simulink model "zad_no_10"  (R2017b)
settings: Solver=VariableStepAuto  StartTime=0.0  StopTime=40  RelTol=1e-3
undefined symbols (not defined in the file): Tp, u_c
settings Model: Creator=micha  LastModifiedBy=micha

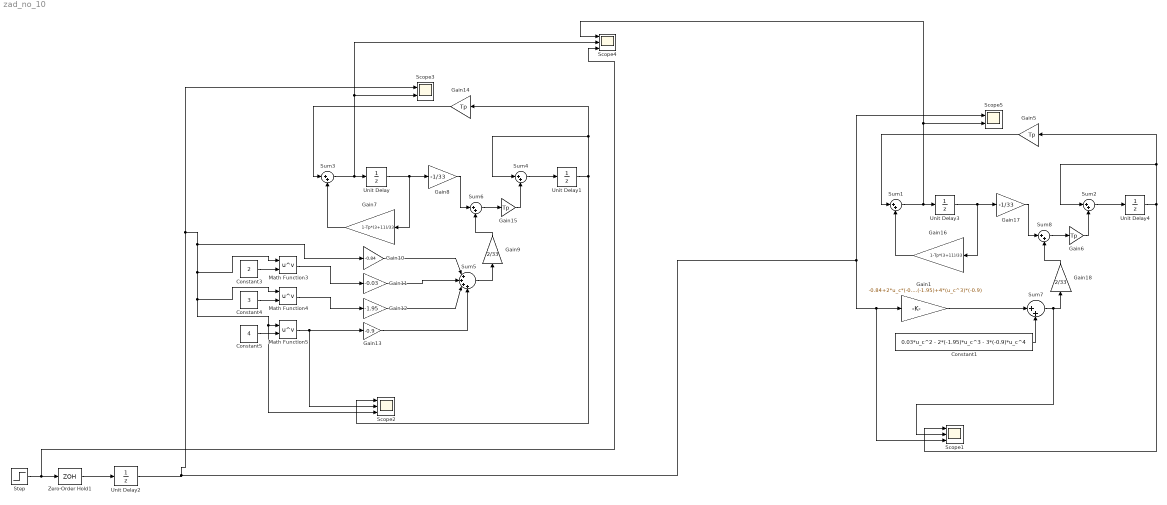
== system zad_no_10 ==
  Constant1 : Constant  Value=0.03*u_c^2 - 2*(-1.95)*u_c^3 - 3*(-0.9)*u_c^4
  Constant3 : Constant  Value=2
  Constant4 : Constant  Value=3
  Constant5 : Constant  Value=4
  Gain1 : Gain  Gain=-0.84+2*u_c*(-0.03)+3*(u_c^2)*(-1.95)+4*(u_c^3)*(-0.9)
  Gain10 : Gain  Gain=-0.84
  Gain11 : Gain  Gain=-0.03
  Gain12 : Gain  Gain=-1.95
  Gain13 : Gain  Gain=-0.9
  Gain14 : Gain  Gain=Tp  ParamDataTypeStr=double
  Gain15 : Gain  Gain=Tp
  Gain16 : Gain  Gain=1-Tp*(3+11)/33  ParamDataTypeStr=double
  Gain17 : Gain  Gain=-1/33
  Gain18 : Gain  Gain=2/33
  Gain5 : Gain  Gain=Tp  ParamDataTypeStr=double
  Gain6 : Gain  Gain=Tp
  Gain7 : Gain  Gain=1-Tp*(3+11)/33  ParamDataTypeStr=double
  Gain8 : Gain  Gain=-1/33
  Gain9 : Gain  Gain=2/33
  Math Function3 : Math  Operator=pow  SaturateOnIntegerOverflow=on
  Math Function4 : Math  Operator=pow  SaturateOnIntegerOverflow=on
  Math Function5 : Math  Operator=pow  SaturateOnIntegerOverflow=on
  Scope1 : Scope  NumInputPorts=3
  Scope2 : Scope  NumInputPorts=3
  Scope3 : Scope  NumInputPorts=2
  Scope4 : Scope  NumInputPorts=3
  Scope5 : Scope  NumInputPorts=2
  Step : Step  SampleTime=0
  Sum{1..4,6..8} (7 alike) : Sum  Inputs=|++
  Sum5 : Sum  Inputs=|++++
  Unit Delay{,1..4} (5 alike) : UnitDelay  SampleTime=Tp
  Zero-Order Hold1 : ZeroOrderHold  SampleTime=Tp
  wires:
  Sum4/1 -> Unit Delay1/1
  Constant5/1 -> Math Function5/2
  Gain7/1 -> Sum3/2
  Unit Delay/1 -> Gain8/1, Gain7/1
  Math Function5/1 -> Scope2/2, Gain13/1
  Gain10/1 -> Sum5/1
  Constant4/1 -> Math Function4/2
  Math Function4/1 -> Gain12/1
  Math Function3/1 -> Gain11/1
  Sum3/1 -> Scope3/2, Scope4/2, Unit Delay/1
  Gain12/1 -> Sum5/3
  Gain11/1 -> Sum5/2
  Unit Delay1/1 -> Sum4/1, Gain14/1, Scope2/1
  Constant3/1 -> Math Function3/2
  Gain13/1 -> Sum5/4
  Sum5/1 -> Gain9/1
  Gain14/1 -> Sum3/1
  Gain9/1 -> Sum6/2
  Gain8/1 -> Sum6/1
  Sum6/1 -> Gain15/1
  Gain15/1 -> Sum4/2
  Sum2/1 -> Unit Delay4/1
  Gain1/1 -> Sum7/1
  Constant1/1 -> Sum7/2
  Gain17/1 -> Sum8/1
  Gain16/1 -> Sum1/2
  Gain6/1 -> Sum2/2
  Step/1 -> Scope4/3, Zero-Order Hold1/1
  Unit Delay4/1 -> Sum2/1, Gain5/1, Scope1/1
  Unit Delay3/1 -> Gain17/1, Gain16/1
  Gain5/1 -> Sum1/1
  Sum1/1 -> Scope4/1, Scope5/2, Unit Delay3/1
  Gain18/1 -> Sum8/2
  Sum7/1 -> Scope1/2, Gain18/1
  Sum8/1 -> Gain6/1
  Unit Delay2/1 -> Scope1/3, Gain1/1, Scope5/1, Scope3/1, Gain10/1, Math Function3/1, Math Function4/1, Scope2/3, Math Function5/1
  Zero-Order Hold1/1 -> Unit Delay2/1
